simulink model "Design_Credit_DAB (1)"  (R2022b)
settings: Solver=ode23t  StartTime=0.0  StopTime=10.0  RelTol=1e-3
libraries: spsIGBTDiodeLib x8, spsSeriesRLCBranchLib x5, spsVoltageMeasurementLib x3, spsCurrentMeasurementLib x2, spsDCVoltageSourceLib x1, spsLinearTransformerLib x1, spspowerguiLib x1
settings Model: Creator=mluser  LastModifiedBy=mluser

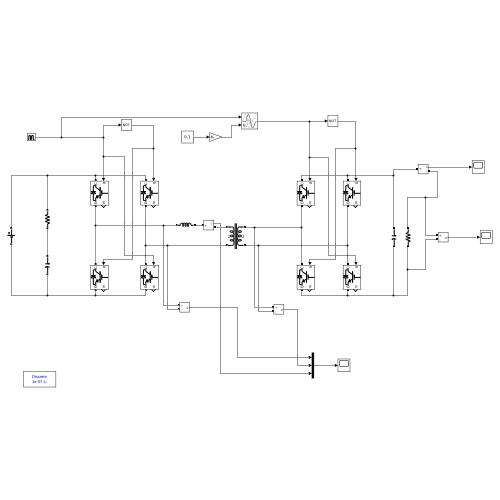
[thumbnail: Simulink's stored preview of the top-level diagram]
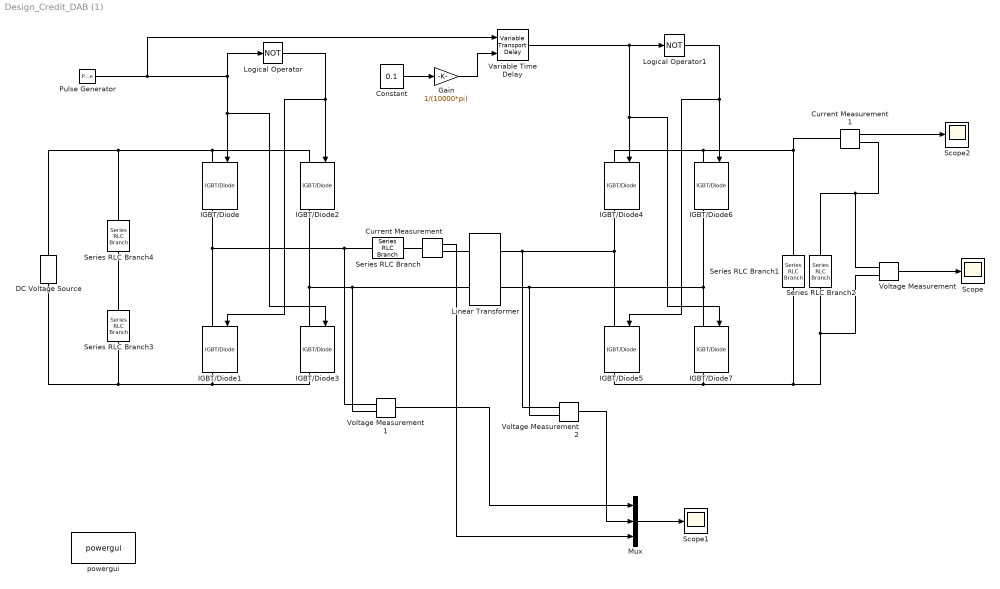
== system Design_Credit_DAB (1) ==
  Constant : Constant  Value=0.1
  Current Measurement : spsCurrentMeasurementLib/Current Measurement  PhasorSimulation=off  OutputType=Complex  PSBequivalent=0
  Current Measurement1 : spsCurrentMeasurementLib/Current Measurement  PhasorSimulation=off  OutputType=Complex  PSBequivalent=0
  DC Voltage Source : spsDCVoltageSourceLib/DC Voltage Source  Amplitude=800  Measurements=None
  Gain : Gain  Gain=1/(10000*pi)
  IGBT/Diode{,1..7} (8 alike) : spsIGBTDiodeLib/IGBT//Diode  Ron=1e-3  Rs=1e5  Cs=inf  Measurements=on
  Linear Transformer : spsLinearTransformerLib/Linear Transformer  UNITS=SI  NominalPower=[ 250e1 1000*pi]  winding1=[300 0 0]  winding2=[250 0 0]  ThreeWindings=off  winding3=[3.15e+05 0.7938 0.084227]  RmLm=[2.0805e3 2866]  Measurements=None  DataType=on
  Logical Operator : Logic  Operator=NOT  AllPortsSameDT=off  OutDataTypeStr=boolean
  Logical Operator1 : Logic  Operator=NOT  AllPortsSameDT=off  OutDataTypeStr=boolean
  Mux : Mux  Inputs=3
  Pulse Generator : DiscretePulseGenerator  PulseType=Time based  Period=1/(10000*pi)  PulseWidth=50
  Scope : Scope
  Scope1 : Scope
  Scope2 : Scope
  Series RLC Branch : spsSeriesRLCBranchLib/Series RLC Branch  LConnTagsString=__new0  RConnTagsString=__new0  BranchType=L  Resistance=1  Inductance=0.102e-3  SetiL0=off  InitialCurrent=0  Capacitance=1e-6  Setx0=off  InitialVoltage=0  Measurements=None
  Series RLC Branch1 : spsSeriesRLCBranchLib/Series RLC Branch  LConnTagsString=__new0  RConnTagsString=__new0  BranchType=C  Resistance=1  Inductance=0.135e-3  SetiL0=off  InitialCurrent=0  Capacitance=50e-6  Setx0=off  InitialVoltage=0  Measurements=None
  Series RLC Branch2 : spsSeriesRLCBranchLib/Series RLC Branch  LConnTagsString=__new0  RConnTagsString=__new0  BranchType=R  Resistance=18  Inductance=0.135e-3  SetiL0=off  InitialCurrent=0  Capacitance=1e-6  Setx0=off  InitialVoltage=0  Measurements=None
  Series RLC Branch3 : spsSeriesRLCBranchLib/Series RLC Branch  LConnTagsString=__new0  RConnTagsString=__new0  BranchType=C  Resistance=1  Inductance=0.135e-3  SetiL0=off  InitialCurrent=0  Capacitance=50e-6  Setx0=off  InitialVoltage=0  Measurements=None
  Series RLC Branch4 : spsSeriesRLCBranchLib/Series RLC Branch  LConnTagsString=__new0  RConnTagsString=__new0  BranchType=R  Resistance=5  Inductance=0.135e-3  SetiL0=off  InitialCurrent=0  Capacitance=1e-6  Setx0=off  InitialVoltage=0  Measurements=None
  Variable Time Delay : VariableTransportDelay  MaximumDelay=10
  Voltage Measurement : spsVoltageMeasurementLib/Voltage Measurement  PhasorSimulation=off  OutputType=Complex  PSBequivalent=0
  Voltage Measurement1 : spsVoltageMeasurementLib/Voltage Measurement  PhasorSimulation=off  OutputType=Complex  PSBequivalent=0
  Voltage Measurement2 : spsVoltageMeasurementLib/Voltage Measurement  PhasorSimulation=off  OutputType=Complex  PSBequivalent=0
  powergui : spspowerguiLib/powergui  Priority=1  SimulationMode=Discrete  SampleTime=1e-7  frequency=60  Iterations=50  frequencyindice=0  Pbase=100e6  ErrMax=1e-4  UnitsV=kV  UnitsW=MW  buscounter=0  FunctionMessages=off  echomessages=off  EnableUseOfTLC=off  CurrentSourceSwitches=off  DisableSnubberDevices=off  DisableRonSwitches=off  DisableVfSwitches=off  DisplayEquations=off  AutomaticDiscreteSolvers=off  SolverType=Tustin/Backward Euler (TBE)  Interpol=off  ExternalGateDelay=off  methode=off  Ts=100  x0status=blocks  SPID=on  SwTol=0  HookPort=off  NonlinearTolerance=1e-4  nMaxIteration=100  ContinueOnMaxIteration=off  RestoreLinks=warning  ResistiveCurrentMeasurement=off  Frange=[0:2:500]  Ylog=off  Xlog=on  ShowGrid=off  save=off  variable=ZData  structure=0  ZoomFFT=off  StartTime=0.0  cycles=1  DisplayStyle=1  fundamental=60  FreqAxis=off  MaxFrequency=1000  frequencyindicesteady=1  RmsSteady=1  display=off
  wires:
  Pulse Generator/1 -> Variable Time Delay/1, Logical Operator/1, IGBT/Diode3/1, IGBT/Diode/1
  Logical Operator/1 -> IGBT/Diode1/1, IGBT/Diode2/1
  Gain/1 -> Variable Time Delay/2
  Variable Time Delay/1 -> Logical Operator1/1, IGBT/Diode7/1, IGBT/Diode4/1
  Logical Operator1/1 -> IGBT/Diode5/1, IGBT/Diode6/1
  Constant/1 -> Gain/1
  Voltage Measurement/1 -> Scope/1
  Current Measurement/1 -> Mux/3
  Voltage Measurement2/1 -> Mux/2
  Voltage Measurement1/1 -> Mux/1
  Mux/1 -> Scope1/1
  Current Measurement1/1 -> Scope2/1
  connections:
  IGBT/Diode/RConn1 -- Voltage Measurement1/LConn1 -- Series RLC Branch/LConn1 -- IGBT/Diode1/LConn1
  IGBT/Diode2/RConn1 -- Voltage Measurement1/LConn2 -- Linear Transformer/LConn2 -- IGBT/Diode3/LConn1
  DC Voltage Source/RConn1 -- Series RLC Branch4/LConn1 -- IGBT/Diode2/LConn1 -- IGBT/Diode/LConn1
  DC Voltage Source/LConn1 -- Series RLC Branch3/RConn1 -- IGBT/Diode3/RConn1 -- IGBT/Diode1/RConn1
  Current Measurement/LConn1 -- Series RLC Branch/RConn1
  Current Measurement/RConn1 -- Linear Transformer/LConn1
  IGBT/Diode4/RConn1 -- Voltage Measurement2/LConn1 -- Linear Transformer/RConn1 -- IGBT/Diode5/LConn1
  IGBT/Diode6/RConn1 -- Voltage Measurement2/LConn2 -- Linear Transformer/RConn2 -- IGBT/Diode7/LConn1
  Voltage Measurement/LConn1 -- Series RLC Branch2/LConn1 -- Current Measurement1/RConn1
  IGBT/Diode5/RConn1 -- Voltage Measurement/LConn2 -- Series RLC Branch2/RConn1 -- Series RLC Branch1/RConn1 -- IGBT/Diode7/RConn1
  Series RLC Branch4/RConn1 -- Series RLC Branch3/LConn1
  Series RLC Branch1/LConn1 -- Current Measurement1/LConn1 -- IGBT/Diode4/LConn1 -- IGBT/Diode6/LConn1
